simulink model "Mophong2"  (R2023a)
settings: Solver=VariableStepAuto  StartTime=0.0  StopTime=10.0  RelTol=1e-3
values from neighbouring files (symbols this model uses):
  Kp2 = cp2*wL    [Code.m]
  Kv2 = cv2*wL    [Code.m]
  position = 7    [Code.m]
  velocity = 7    [Code.m]
libraries: simulink x1
settings Model: Creator=admin  LastModifiedBy=admin

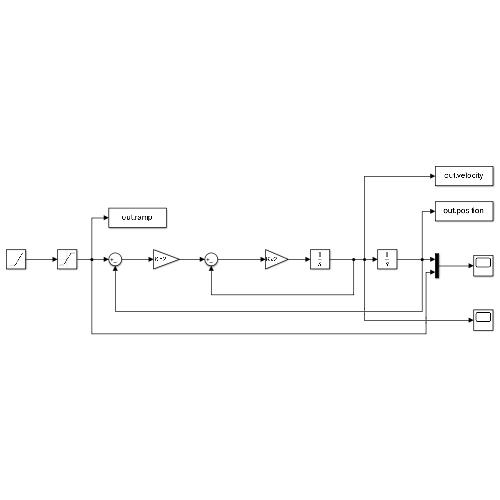
[thumbnail: Simulink's stored preview of the top-level diagram]
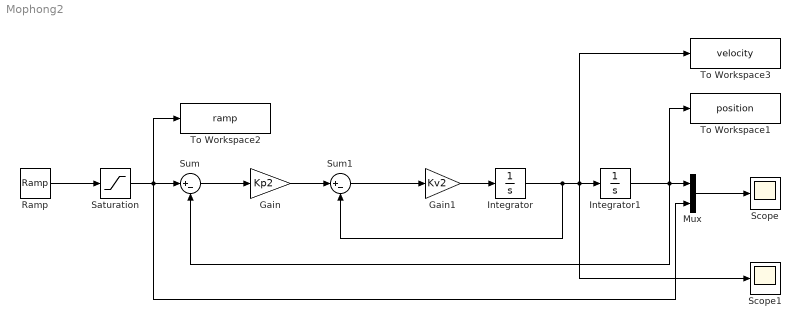
== system Mophong2 ==
  Gain : Gain  Gain=Kp2
  Gain1 : Gain  Gain=Kv2
  Integrator : Integrator
  Integrator1 : Integrator
  Mux : Mux  Inputs=2
  Ramp : simulink/Sources/Ramp  slope=velocity  start=0  InitialOutput=0
  Saturation : Saturate  UpperLimit=position  LowerLimit=0
  Scope : Scope
  Scope1 : Scope
  Sum : Sum  Inputs=|+-
  Sum1 : Sum  Inputs=|+-
  To Workspace1 : ToWorkspace  VariableName=position  SaveFormat=Timeseries  SampleTime=-1
  To Workspace2 : ToWorkspace  VariableName=ramp  SaveFormat=Timeseries  SampleTime=-1
  To Workspace3 : ToWorkspace  VariableName=velocity  SaveFormat=Timeseries  SampleTime=-1
  wires:
  Ramp/1 -> Saturation/1
  Saturation/1 -> Mux/2, To Workspace2/1, Sum/1
  Sum/1 -> Gain/1
  Gain/1 -> Sum1/1
  Sum1/1 -> Gain1/1
  Gain1/1 -> Integrator/1
  Integrator/1 -> Sum1/2, To Workspace3/1, Scope1/1, Integrator1/1
  Integrator1/1 -> Mux/1, To Workspace1/1, Sum/2
  Mux/1 -> Scope/1
